simulink model "untitled_restored_from_autosave"  (R2025b)
settings: Solver=VariableStepAuto  StartTime=0.0  StopTime=40  RelTol=1e-3
values from neighbouring files (symbols this model uses):
  accel_bias = [0.05; 0.05; 0.05]    [init_sim_6dof.m]
  alt_bias = [0; 0; 15]    [init_sim_6dof.m]
  Cd_0 = [0.4, 0.42, 0.65, 0.55, 0.45, 0.35, 0.30, 0.28]    [init_sim_6dof.m]
  Cma = [-25, -28, -35,  -40,  -35,  -30,  -25,  -20 ]    [init_sim_6dof.m]
  Cme = -15    [init_sim_6dof.m]
  Cna = [15,  16,   18,   20,   18,   15,   12,   10  ]    [init_sim_6dof.m]
  Cne = -15    [init_sim_6dof.m]
  Empuje_Max = 16000    [init_sim_6dof.m]
  gyro_bias = [0.01; 0.01; 0.01]    [init_sim_6dof.m]
  L_ref = diametro    (= 0.127)    [init_sim_6dof.m]
  lat_0 = 40.4168    [init_sim_6dof.m]
  lon_0 = -3.7038    [init_sim_6dof.m]
  Mach_vec = [0.0, 0.8, 1.0, 1.2, 1.5, 2.0, 3.0, 4.0]    [init_sim_6dof.m]
  masa_ini = 85.0    (= 85)    [init_sim_6dof.m]
  N_pn = 4.0    (= 4)    [init_sim_6dof.m]
  pitch_0 = 0    [init_sim_6dof.m]
  pos_0_ned = [0; 0; -alt_0]    [init_sim_6dof.m]
  pos_target_0 = [10000; 0; -5000]    [init_sim_6dof.m]
  quat_0 = angle2quat(yaw_0, pitch_0, roll_0, 'ZYX')'    [init_sim_6dof.m]
  roll_0 = 0    [init_sim_6dof.m]
  S_ref = pi*(diametro/2)^2    (= 0.0126676869774)    [init_sim_6dof.m]
  t_burn = 5.0    (= 5)    [init_sim_6dof.m]
  Ts = 0.005    [init_sim_6dof.m]
  Ts_gnss = 0.1    [init_sim_6dof.m]
  vel_target_0 = [-250; 0; 0]    [init_sim_6dof.m]
  yaw_0 = 0    [init_sim_6dof.m]
undefined symbols (not defined in the file or in its folder): Accel_Body, magnitude, Omega_Body, Pos_NED
libraries: simulink x5, slpidlib x2, aerolibasang x2, aerolibanim x1, aerolibatmos2 x1
settings Model: Creator=Pc  LastModifiedBy=Pc

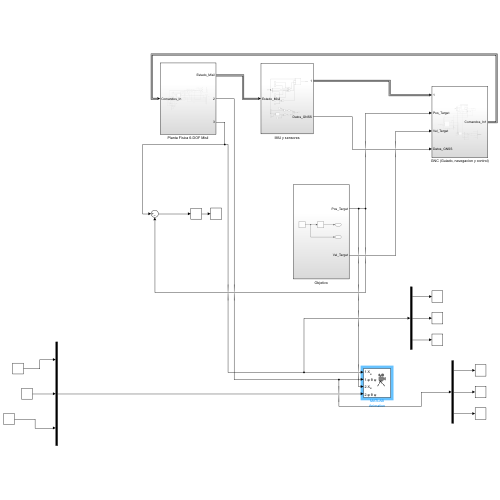
[thumbnail: Simulink's stored preview of the top-level diagram]
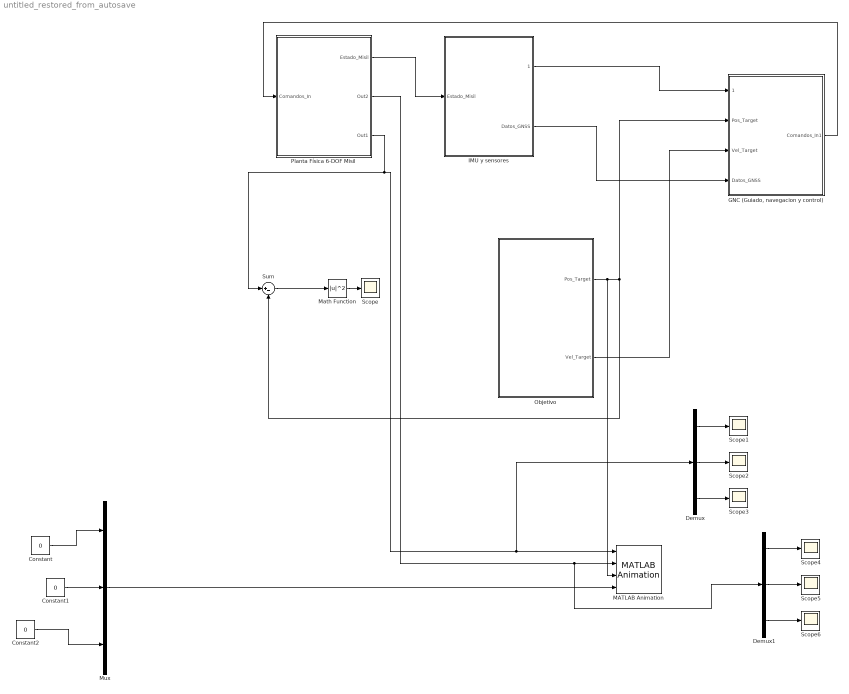
== system untitled_restored_from_autosave ==
  Constant : Constant  Value=0
  Constant1 : Constant  Value=0
  Constant2 : Constant  Value=0
  Demux : Demux  Outputs=3
  Demux1 : Demux  Outputs=3
  "GNC (Guiado, navegacion y control)" : Subsystem
  IMU y sensores : Subsystem
  MATLAB Animation : aerolibanim/MATLAB Animation  Tag=Matlab Animation 6 DOF  Vehicles=2  Geometries={'testrocket.ac', 'pa24-250_orange.ac'}  BoundingBoxCoordinates=[-50,50,-50,50,-50,50]  CameraOffset=[-150,-50,0]  CameraViewAngle=50  SampleTime=0.05  FigurePosition=[-248,-120,605,515]
  Math Function : Math  Operator=magnitude^2
  Mux : Mux  Inputs=3
  Objetivo : Subsystem
  Planta Física 6-DOF Misil : Subsystem
  Scope{,1..6} (7 alike) : Scope
      Scope settings: ActiveDisplayYMinimum=-2.9498159445716068E+7  ActiveDisplayYMaximum=4.0106517826440394E+7
      Scope1 settings: ActiveDisplayYMinimum=-21.388722849455736  ActiveDisplayYMaximum=29.150281058057079  DataLoggingVariableName=ScopeData2
      Scope2 settings: DataLoggingVariableName=ScopeData3
      Scope3 settings: ActiveDisplayYMinimum=-15.325503543946462  ActiveDisplayYMaximum=15.701060775623862  DataLoggingVariableName=ScopeData4
      Scope4 settings: ActiveDisplayYMinimum=-2.4693491349201278  ActiveDisplayYMaximum=1.7034269315097514  DataLoggingVariableName=ScopeData5
      Scope5 settings: ActiveDisplayYMinimum=-1.9297866797423937  ActiveDisplayYMaximum=2.0089780542618731  DataLoggingVariableName=ScopeData6
      Scope6 settings: ActiveDisplayYMinimum=-1  ActiveDisplayYMaximum=1  DataLoggingVariableName=ScopeData7
  Sum : Sum  Inputs=|+-
  wires:
  Planta Física 6-DOF Misil/1(Estado_Misil) -> IMU y sensores/1(Estado_Misil)
  IMU y sensores/1(1) -> "GNC (Guiado, navegacion y control)"/1(1)
  Objetivo/1(Pos_Target) -> MATLAB Animation/3, Sum/2, "GNC (Guiado, navegacion y control)"/2(Pos_Target)
  Objetivo/2(Vel_Target) -> "GNC (Guiado, navegacion y control)"/3(Vel_Target)
  "GNC (Guiado, navegacion y control)"/1(Comandos_In1) -> Planta Física 6-DOF Misil/1(Comandos_In)
  Sum/1 -> Math Function/1
  Math Function/1 -> Scope/1
  IMU y sensores/2(Datos_GNSS) -> "GNC (Guiado, navegacion y control)"/4(Datos_GNSS)
  Planta Física 6-DOF Misil/2(Out2) -> Demux1/1, MATLAB Animation/2
  Constant2/1 -> Mux/3
  Constant1/1 -> Mux/2
  Constant/1 -> Mux/1
  Mux/1 -> MATLAB Animation/4
  Planta Física 6-DOF Misil/3(Out1) -> Sum/1, Demux/1, MATLAB Animation/1
  Demux1/3 -> Scope6/1
  Demux1/2 -> Scope5/1
  Demux1/1 -> Scope4/1
  Demux/3 -> Scope3/1
  Demux/2 -> Scope2/1
  Demux/1 -> Scope1/1

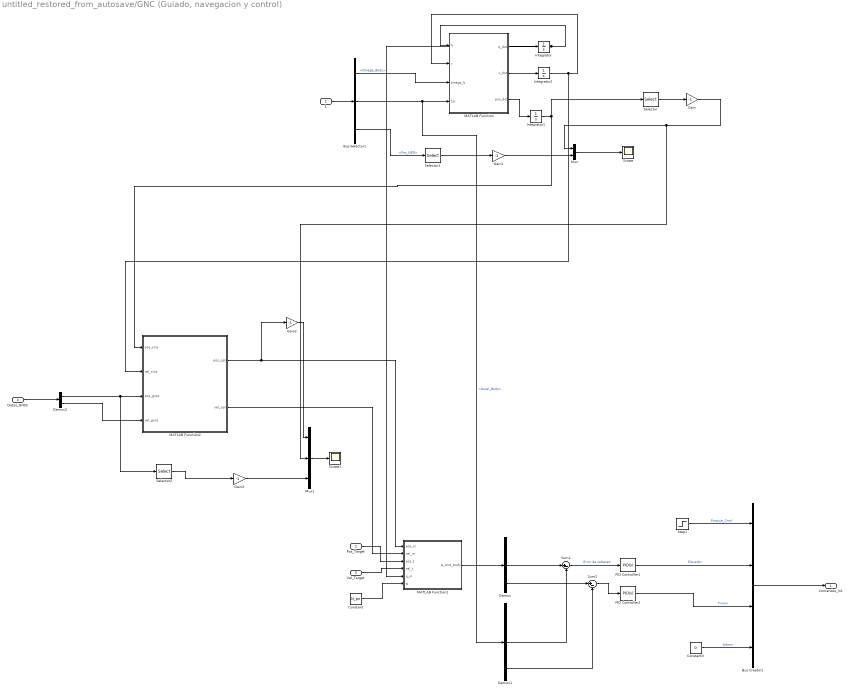
== system untitled_restored_from_autosave/GNC (Guiado, navegacion y control) ==
  1 : Inport  OutDataTypeStr=Bus: Bus_Estado
  Pos_Target : Inport  Port=2
  Vel_Target : Inport  Port=3
  Datos_GNSS : Inport  Port=4
  Bus Creator1 : BusCreator  Inputs=4  OutDataTypeStr=Bus: Bus_Comandos
  Bus Selector1 : BusSelector  OutputSignals=Omega_Body,Accel_Body,Pos_NED
  Constant : Constant  Value=N_pn
  Constant3 : Constant  Value=0
  Demux : Demux  Outputs=3
  Demux1 : Demux  Outputs=3
  Demux2 : Demux  Outputs=2
  Gain{,1..3} (4 alike) : Gain  Gain=-1
  Integrator : Integrator  InitialCondition=quat_0
  Integrator1 : Integrator  InitialCondition=pos_0_ned
  Integrator2 : Integrator  InitialCondition=[250; 0; 0]
  MATLAB Function : MATLAB Function  TreatAsAtomicUnit=on
  MATLAB Function1 : MATLAB Function  TreatAsAtomicUnit=on
  MATLAB Function2 : MATLAB Function  TreatAsAtomicUnit=on
  Mux : Mux  Inputs=2
  Mux1 : Mux  Inputs=3
  PID Controller1 : slpidlib/PID Controller  Controller=PID  Form=Parallel  TimeDomain=Continuous-time  UseExternalTs=off  SampleTime=-1  IntegratorMethod=Forward Euler  FilterMethod=Forward Euler  ControllerParametersSource=internal  P=0.05  I=0.01  UseKiTs=off  D=0  UseExternalDerivativeSource=off  N=100  UseFilter=on  TunerSelectOption=Transfer Function Based (PID Tuner App)  InitialConditionSource=internal  InitialConditionForIntegrator=0  InitialConditionForFilter=0  DifferentiatorICPrevScaledInput=0  ExternalReset=none  TrackingMode=off  Kt=1  LimitOutput=on  SatLimitsSource=internal  UpperSaturationLimit=0.5  LowerSaturationLimit=-0.5  LinearizeAsGain=on  AntiWindupMode=none  Kb=1  LimitIntegrator=off  UpperIntegratorSaturationLimit=inf  LowerIntegratorSaturationLimit=-inf  POutMin=[]  POutMax=[]  IOutMin=[]  IOutMax=[]  DOutMin=[]  DOutMax=[]  NOutMin=[]  NOutMax=[]  SumOutMin=[]  SumOutMax=[]  SaturationOutMin=[]  SaturationOutMax=[]  PParamMin=[]  PParamMax=[]  IParamMin=[]  IParamMax=[]  DParamMin=[]  DParamMax=[]  NParamMin=[]  NParamMax=[]  KbParamMin=[]  KbParamMax=[]  KtParamMin=[]  KtParamMax=[]  KbOutMin=[]  KbOutMax=[]  KtOutMin=[]  KtOutMax=[]  IntegratorOutMin=[]  IntegratorOutMax=[]  FilterOutMin=[]  FilterOutMax=[]  SumI1OutMin=[]  SumI1OutMax=[]  SumI2OutMin=[]  SumI2OutMax=[]  SumI3OutMin=[]  SumI3OutMax=[]  SumI4OutMin=[]  SumI4OutMax=[]  SumDOutMin=[]  SumDOutMax=[]  DifferentiatorOutMin=[]  DifferentiatorOutMax=[]  FilterDiffOutCoefMin=[]  FilterDiffOutCoefMax=[]  ReciprocalOutMin=[]  ReciprocalOutMax=[]  SumDenOutMin=[]  SumDenOutMax=[]  SumNumOutMin=[]  SumNumOutMax=[]  DivideOutMin=[]  DivideOutMax=[]  UdiffTsProdOutMin=[]  UdiffTsProdOutMax=[]  NTsProdOutMin=[]  NTsProdOutMax=[]  UintegralTsProdOutMin=[]  UintegralTsProdOutMax=[]  UngainTsProdOutMin=[]  UngainTsProdOutMax=[]  ClampingZeroOutDataTypeStr=Inherit: Inherit via back propagation  ClampingZeroOutMin=[]  ClampingZeroOutMax=[]  FilterDenConstantOutDataTypeStr=Inherit: Inherit via back propagation  FilterDenConstantOutMin=[]  FilterDenConstantOutMax=[]  PCopyOutDataTypeStr=Inherit: Inherit via back propagation  PCopyOutMin=[]  PCopyOutMax=[]  NCopyOutDataTypeStr=Inherit: Inherit via back propagation  NCopyOutMin=[]  NCopyOutMax=[]  IntegratorContinuousStateAttributes=''  IntegratorStateMustResolveToSignalObject=off  IntegratorRTWStateStorageClass=Auto  FilterContinuousStateAttributes=''  FilterStateMustResolveToSignalObject=off  FilterRTWStateStorageClass=Auto  ParallelPVariant=InternalParameters  IdealPVariant=Disabled  IVariant=InternalParameters  DVariant=InternalParameters  IntegratorVariant=Continuous  SatVariant=Enabled  AWVariant=Passthrough  PCopyVariant=Disabled  TRVariant=Disabled  FdbkBlocksVariant=Forward  IdealPFdbkVariant=Disabled  SatFdbkVariant=Disabled  DerivativeFilterVariant=ContFilter  NVariant=InternalParameters  NCopyVariant=Disabled  FilterICVariant=InternalICsFilter  IntegratorICVariant=InternalICs  ExternalResetVariant=Disabled  TRSumVariant=Passthrough  SumFdbkVariant=Disabled  SumVariant=Sum_PID  TsampFilterVariant=InternalTs  TsampNgainVariant=Passthrough  TsampIntegralVariant=Disabled_SignalSpec  ExternalSaturationOutDataTypeStr=Inherit: Same as second input  DerivativeSourceVariant=ErrorSignal  PreIntVariant=InternalPreInt
  PID Controller2 : slpidlib/PID Controller  Controller=PID  Form=Parallel  TimeDomain=Continuous-time  UseExternalTs=off  SampleTime=-1  IntegratorMethod=Forward Euler  FilterMethod=Forward Euler  ControllerParametersSource=internal  P=0.05  I=0.01  UseKiTs=off  D=0  UseExternalDerivativeSource=off  N=100  UseFilter=on  TunerSelectOption=Transfer Function Based (PID Tuner App)  InitialConditionSource=internal  InitialConditionForIntegrator=0  InitialConditionForFilter=0  DifferentiatorICPrevScaledInput=0  ExternalReset=none  TrackingMode=off  Kt=1  LimitOutput=on  SatLimitsSource=internal  UpperSaturationLimit=0.5  LowerSaturationLimit=-0.5  LinearizeAsGain=on  AntiWindupMode=none  Kb=1  LimitIntegrator=off  UpperIntegratorSaturationLimit=inf  LowerIntegratorSaturationLimit=-inf  POutMin=[]  POutMax=[]  IOutMin=[]  IOutMax=[]  DOutMin=[]  DOutMax=[]  NOutMin=[]  NOutMax=[]  SumOutMin=[]  SumOutMax=[]  SaturationOutMin=[]  SaturationOutMax=[]  PParamMin=[]  PParamMax=[]  IParamMin=[]  IParamMax=[]  DParamMin=[]  DParamMax=[]  NParamMin=[]  NParamMax=[]  KbParamMin=[]  KbParamMax=[]  KtParamMin=[]  KtParamMax=[]  KbOutMin=[]  KbOutMax=[]  KtOutMin=[]  KtOutMax=[]  IntegratorOutMin=[]  IntegratorOutMax=[]  FilterOutMin=[]  FilterOutMax=[]  SumI1OutMin=[]  SumI1OutMax=[]  SumI2OutMin=[]  SumI2OutMax=[]  SumI3OutMin=[]  SumI3OutMax=[]  SumI4OutMin=[]  SumI4OutMax=[]  SumDOutMin=[]  SumDOutMax=[]  DifferentiatorOutMin=[]  DifferentiatorOutMax=[]  FilterDiffOutCoefMin=[]  FilterDiffOutCoefMax=[]  ReciprocalOutMin=[]  ReciprocalOutMax=[]  SumDenOutMin=[]  SumDenOutMax=[]  SumNumOutMin=[]  SumNumOutMax=[]  DivideOutMin=[]  DivideOutMax=[]  UdiffTsProdOutMin=[]  UdiffTsProdOutMax=[]  NTsProdOutMin=[]  NTsProdOutMax=[]  UintegralTsProdOutMin=[]  UintegralTsProdOutMax=[]  UngainTsProdOutMin=[]  UngainTsProdOutMax=[]  ClampingZeroOutDataTypeStr=Inherit: Inherit via back propagation  ClampingZeroOutMin=[]  ClampingZeroOutMax=[]  FilterDenConstantOutDataTypeStr=Inherit: Inherit via back propagation  FilterDenConstantOutMin=[]  FilterDenConstantOutMax=[]  PCopyOutDataTypeStr=Inherit: Inherit via back propagation  PCopyOutMin=[]  PCopyOutMax=[]  NCopyOutDataTypeStr=Inherit: Inherit via back propagation  NCopyOutMin=[]  NCopyOutMax=[]  IntegratorContinuousStateAttributes=''  IntegratorStateMustResolveToSignalObject=off  IntegratorRTWStateStorageClass=Auto  FilterContinuousStateAttributes=''  FilterStateMustResolveToSignalObject=off  FilterRTWStateStorageClass=Auto  ParallelPVariant=InternalParameters  IdealPVariant=Disabled  IVariant=InternalParameters  DVariant=InternalParameters  IntegratorVariant=Continuous  SatVariant=Enabled  AWVariant=Passthrough  PCopyVariant=Disabled  TRVariant=Disabled  FdbkBlocksVariant=Forward  IdealPFdbkVariant=Disabled  SatFdbkVariant=Disabled  DerivativeFilterVariant=ContFilter  NVariant=InternalParameters  NCopyVariant=Disabled  FilterICVariant=InternalICsFilter  IntegratorICVariant=InternalICs  ExternalResetVariant=Disabled  TRSumVariant=Passthrough  SumFdbkVariant=Disabled  SumVariant=Sum_PID  TsampFilterVariant=InternalTs  TsampNgainVariant=Passthrough  TsampIntegralVariant=Disabled_SignalSpec  ExternalSaturationOutDataTypeStr=Inherit: Same as second input  DerivativeSourceVariant=ErrorSignal  PreIntVariant=InternalPreInt
  Scope : Scope
      settings: ActiveDisplayYMinimum=-3409.6489857780471  ActiveDisplayYMaximum=9919.0359935642336
  Scope1 : Scope
      settings: ActiveDisplayYMinimum=-14494.057795394729  ActiveDisplayYMaximum=13064.034716970949
  Selector : Selector  InputPortWidth=3  IndexOptions=Index vector (dialog)  Indices=3  OutputSizes=1
  Selector1 : Selector  InputPortWidth=3  IndexOptions=Index vector (dialog)  Indices=3  OutputSizes=1
  Selector2 : Selector  InputPortWidth=3  IndexOptions=Index vector (dialog)  Indices=3  OutputSizes=1
  Step1 : Step  Time=t_burn  Before=Empuje_Max  After=0  SampleTime=0
  Sum1 : Sum  Inputs=|+-
  Sum2 : Sum  Inputs=|+-
  Comandos_In1 : Outport
  wires:
  Selector/1 -> Gain/1
  Gain/1 -> Mux1/2, Mux/1
  1/1 -> Bus Selector1/1
  MATLAB Function/1(q_dot) -> Integrator/1
  MATLAB Function/2(v_dot) -> Integrator2/1
  MATLAB Function/3(pos_dot) -> Integrator1/1
  Integrator/1 -> MATLAB Function/1(q), MATLAB Function1/5(q_m)
  Integrator2/1 -> MATLAB Function2/2(vel_sins), MATLAB Function/2(v)
  Bus Selector1/1 -> MATLAB Function/3(omega_b)  "<Omega_Body>"
  Bus Selector1/2 -> Demux1/1, MATLAB Function/4(f_b)  "<Accel_Body>"
  Integrator1/1 -> Selector/1, MATLAB Function2/1(pos_sins)
  Gain1/1 -> Mux/2
  Selector1/1 -> Gain1/1
  Bus Selector1/3 -> Selector1/1  "<Pos_NED>"
  Mux/1 -> Scope/1
  Pos_Target/1 -> MATLAB Function1/3(pos_t)
  Vel_Target/1 -> MATLAB Function1/4(vel_t)
  Constant/1 -> MATLAB Function1/6(N)
  MATLAB Function1/1(A_cmd_body) -> Demux/1
  Demux/2 -> Sum1/1
  Demux1/2 -> Sum1/2
  Sum1/1 -> PID Controller1/1  "Error de cabeceo"
  PID Controller1/1 -> Bus Creator1/2  "Elevador"
  Demux/3 -> Sum2/1
  Demux1/3 -> Sum2/2
  Sum2/1 -> PID Controller2/1
  PID Controller2/1 -> Bus Creator1/3  "Timon"
  Step1/1 -> Bus Creator1/1  "Empuje_Cmd"
  Constant3/1 -> Bus Creator1/4  "Aleron"
  Bus Creator1/1 -> Comandos_In1/1
  Datos_GNSS/1 -> Demux2/1
  Demux2/1 -> Selector2/1, MATLAB Function2/3(pos_gnss)
  Demux2/2 -> MATLAB Function2/4(vel_gnss)
  MATLAB Function2/1(pos_opt) -> Gain2/1, MATLAB Function1/1(pos_m)
  MATLAB Function2/2(vel_opt) -> MATLAB Function1/2(vel_m)
  Gain2/1 -> Mux1/1
  Mux1/1 -> Scope1/1
  Selector2/1 -> Gain3/1
  Gain3/1 -> Mux1/3

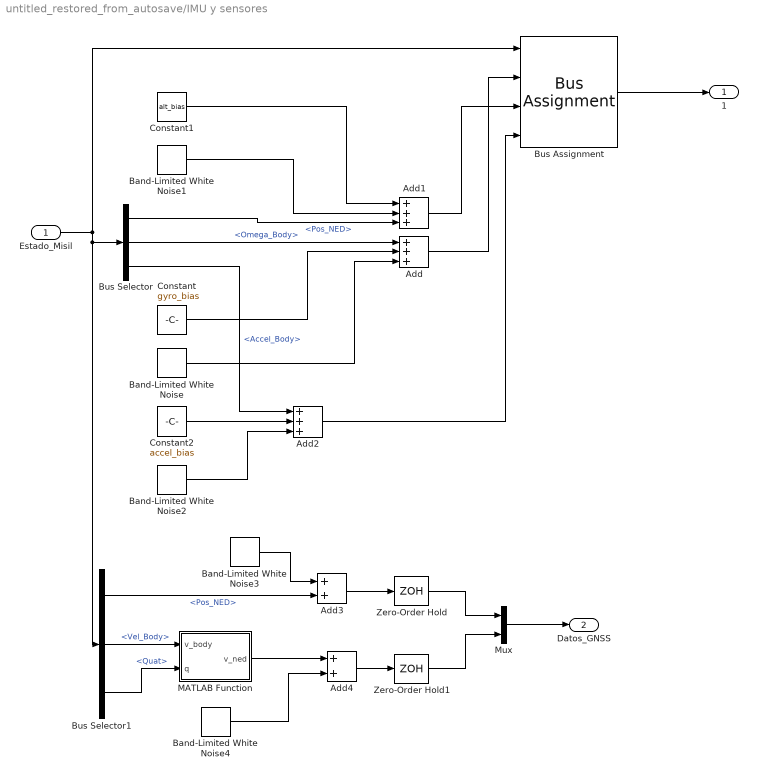
== system untitled_restored_from_autosave/IMU y sensores ==
  Estado_Misil : Inport  OutDataTypeStr=Bus: Bus_Estado
  Add : Sum  Inputs=+++
  Add1 : Sum  Inputs=+++
  Add2 : Sum  Inputs=+++
  Add3 : Sum
  Add4 : Sum
  Band-Limited White Noise : simulink/Sources/Band-Limited White Noise  Cov=gyro_noise_power  Ts=Ts  seed=[23341]
  Band-Limited White Noise1 : simulink/Sources/Band-Limited White Noise  Cov=alt_noise_power  Ts=Ts  seed=[23341]
  Band-Limited White Noise2 : simulink/Sources/Band-Limited White Noise  Cov=accel_noise_power  Ts=Ts  seed=[23341]
  Band-Limited White Noise3 : simulink/Sources/Band-Limited White Noise  Cov=gnss_noise_pos  Ts=Ts_gnss  seed=[23341]
  Band-Limited White Noise4 : simulink/Sources/Band-Limited White Noise  Cov=gnss_noise_vel  Ts=Ts_gnss  seed=[23341]
  Bus Assignment : BusAssignment  AssignedSignals=Omega_Body,Pos_NED,Accel_Body
  Bus Selector : BusSelector  OutputSignals=Pos_NED,Omega_Body,Accel_Body
  Bus Selector1 : BusSelector  OutputSignals=Pos_NED,Vel_Body,Quat
  Constant : Constant  Value=gyro_bias
  Constant1 : Constant  Value=alt_bias
  Constant2 : Constant  Value=accel_bias
  MATLAB Function : MATLAB Function  TreatAsAtomicUnit=on
  Mux : Mux  Inputs=2
  Zero-Order Hold : ZeroOrderHold  SampleTime=Ts_gnss
  Zero-Order Hold1 : ZeroOrderHold  SampleTime=Ts_gnss
  1 : Outport  OutDataTypeStr=Bus: Bus_Estado
  Datos_GNSS : Outport  Port=2
  wires:
  Bus Selector/2 -> Add/1  "<Omega_Body>"
  Constant/1 -> Add/2
  Band-Limited White Noise/1 -> Add/3
  Bus Selector/1 -> Add1/3  "<Pos_NED>"
  Band-Limited White Noise1/1 -> Add1/2
  Constant1/1 -> Add1/1
  Add/1 -> Bus Assignment/2
  Add1/1 -> Bus Assignment/3
  Bus Assignment/1 -> 1/1
  Bus Selector/3 -> Add2/1  "<Accel_Body>"
  Constant2/1 -> Add2/2
  Band-Limited White Noise2/1 -> Add2/3
  Add2/1 -> Bus Assignment/4
  Estado_Misil/1 -> Bus Selector1/1, Bus Selector/1, Bus Assignment/1
  Bus Selector1/2 -> MATLAB Function/1(v_body)  "<Vel_Body>"
  Bus Selector1/3 -> MATLAB Function/2(q)  "<Quat>"
  Bus Selector1/1 -> Add3/2  "<Pos_NED>"
  Band-Limited White Noise3/1 -> Add3/1
  Add3/1 -> Zero-Order Hold/1
  Add4/1 -> Zero-Order Hold1/1
  MATLAB Function/1(v_ned) -> Add4/1
  Band-Limited White Noise4/1 -> Add4/2
  Zero-Order Hold/1 -> Mux/1
  Zero-Order Hold1/1 -> Mux/2
  Mux/1 -> Datos_GNSS/1

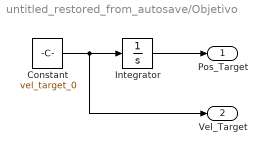
== system untitled_restored_from_autosave/Objetivo ==
  Constant : Constant  Value=vel_target_0
  Integrator : Integrator  InitialCondition=pos_target_0
  Pos_Target : Outport
  Vel_Target : Outport  Port=2
  wires:
  Constant/1 -> Vel_Target/1, Integrator/1
  Integrator/1 -> Pos_Target/1

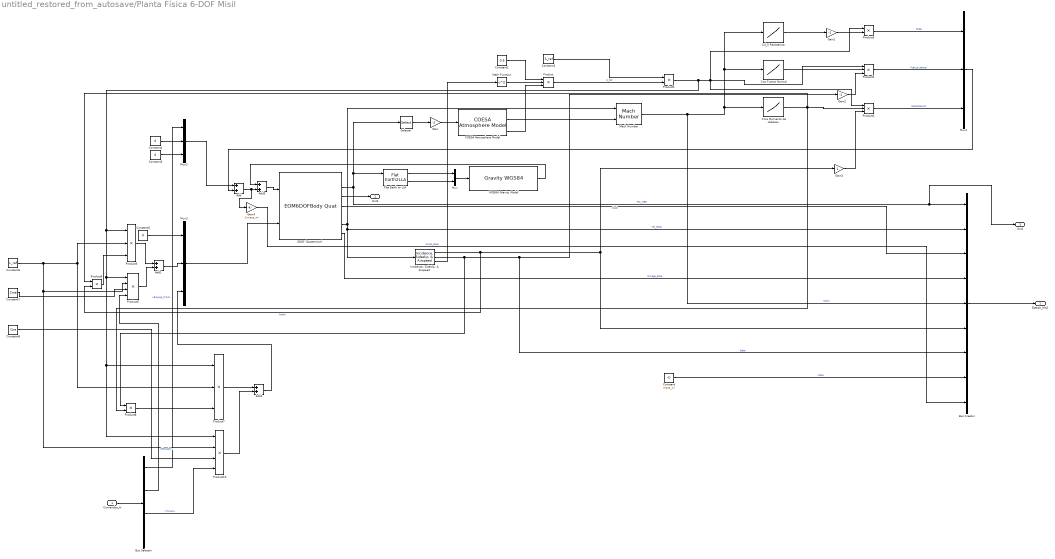
== system untitled_restored_from_autosave/Planta Física 6-DOF Misil ==
  Comandos_In : Inport  OutDataTypeStr=Bus: Bus_Comandos
  6DOF (Quaternion) : EOM6DOFBodyQuat  xme_0=pos_0_ned  Vm_0=vel_0_body  eul_0=[roll_0, pitch_0, yaw_0]  pm_0=omega_0_body  mass_0=masa_ini  inertia=I_tensor
  Add{,1..3} (4 alike) : Sum
  Bus Creator : BusCreator  Inputs=9  OutDataTypeStr=Bus: Bus_Estado
  Bus Selector : BusSelector  OutputSignals=Empuje_Cmd,Elevador,Timon,Aleron
  COESA Atmosphere Model : aerolibatmos2/COESA Atmosphere Model  units=Metric (MKS)  spec=1976 COESA-extended U.S. Standard Atmosphere  model=Profile  profile_var=High temperature  profile_percent=1%  profile_alt=5 km (16404 ft)  envelope_var=High temperature  envelope_percent=1%  action=Warning
  Cd_0 Resistencia : Lookup_n-D  NumberOfTableDimensions=1  BreakpointsForDimension1=Mach_vec  Table=Cd_0  InternalRulePriority=Speed  RndMeth=Simplest
  Cma Momento de cabeceo : Lookup_n-D  NumberOfTableDimensions=1  BreakpointsForDimension1=Mach_vec  Table=Cma  InternalRulePriority=Speed  RndMeth=Simplest
  Cna Fuerza Normal : Lookup_n-D  NumberOfTableDimensions=1  BreakpointsForDimension1=Mach_vec  Table=Cna  InternalRulePriority=Speed  RndMeth=Simplest
  Constant : Constant  Value=masa_ini
  Constant1 : Constant  Value=0.5
  Constant2 : Constant  Value=S_ref
  Constant3 : Constant  Value=0
  Constant4 : Constant  Value=0
  Constant5 : Constant  Value=0
  Constant6 : Constant  Value=L_ref
  Constant7 : Constant  Value=Cme
  Constant8 : Constant  Value=Cne
  Flat Earth to LLA : FlatEarth2LLA  LL0=[lat_0 lon_0]
  Gain : Gain  Gain=-1
  Gain1 : Gain  Gain=-1
  Gain2 : Gain  Gain=-1
  Gain3 : Gain
  Gain4 : Gain  Gain=1/masa_ini
  "Incidence, Sideslip, & Airspeed" : aerolibasang/Incidence, Sideslip, & Airspeed
  Mach Number : aerolibasang/Mach Number
  Math Function : Math  Operator=square
  Mux : Mux  Inputs=2
  Mux1 : Mux  Inputs=3
  Mux2 : Mux  Inputs=3
  Mux3 : Mux  Inputs=3
  Product{,2,4..5,7} (5 alike) : Product  Inputs=3
  Product{1,3,6,8} (4 alike) : Product
  Product10 : Product  Inputs=4
  Product9 : Product  Inputs=4
  Selector : Selector  InputPortWidth=3  IndexOptions=Index vector (dialog)  Indices=3  OutputSizes=1
  "WGS84 Gravity Model  " : GravityWGS84
  Estado_Misil : Outport  OutDataTypeStr=Bus: Bus_Estado
  Out2 : Outport  Port=2
  Out1 : Outport  Port=3
  wires:
  6DOF (Quaternion)/2 -> Out1/1, Bus Creator/1, Selector/1, Flat Earth to LLA/1  "Pos_NED"
  Selector/1 -> Gain/1
  Gain/1 -> COESA Atmosphere Model/1
  Flat Earth to LLA/1 -> Mux/1
  Flat Earth to LLA/2 -> Mux/2
  Mux/1 -> "WGS84 Gravity Model  "/1
  6DOF (Quaternion)/6 -> "Incidence, Sideslip, & Airspeed"/1, Bus Creator/2, Mach Number/1  "Vel_Body"
  COESA Atmosphere Model/2 -> Mach Number/2
  6DOF (Quaternion)/4 -> Bus Creator/3  "Quat"
  6DOF (Quaternion)/7 -> Bus Creator/4  "Omega_Body"
  Mach Number/1 -> Cma Momento de cabeceo/1, Cd_0 Resistencia/1, Cna Fuerza Normal/1, Bus Creator/5  "Mach"
  "Incidence, Sideslip, & Airspeed"/1 -> Product6/2, Gain3/1, Bus Creator/6  "Alpha"
  "Incidence, Sideslip, & Airspeed"/2 -> Product8/1, Gain2/1, Bus Creator/7  "Beta"
  Constant/1 -> Bus Creator/8  "Masa"
  "Incidence, Sideslip, & Airspeed"/3 -> Math Function/1
  Constant1/1 -> Product/1
  Math Function/1 -> Product/2
  COESA Atmosphere Model/4 -> Product/3
  Constant2/1 -> Product1/1
  Product/1 -> Product1/2  "q_bar"
  Cd_0 Resistencia/1 -> Gain1/1
  Product1/1 -> Product10/1, Product7/1, Product9/1, Product5/1, Product4/1, Product3/1, Product2/1
  Cna Fuerza Normal/1 -> Product2/2
  Gain2/1 -> Product2/3
  Gain1/1 -> Product3/2
  Cma Momento de cabeceo/1 -> Product8/2, Product6/1, Product4/2
  Gain3/1 -> Product4/3
  Product2/1 -> Mux1/2  "Fuerza Lateral"
  Product3/1 -> Mux1/1  "Drag"
  Product4/1 -> Mux1/3  "Sustentación"
  Constant4/1 -> Mux2/2
  Constant3/1 -> Mux2/3
  Mux1/1 -> Add/2
  Constant5/1 -> Mux3/1
  Constant6/1 -> Product10/2, Product9/2, Product7/2, Product5/2
  Product6/1 -> Product5/3
  Product8/1 -> Product7/3
  Mux3/1 -> 6DOF (Quaternion)/2
  Comandos_In/1 -> Bus Selector/1
  Bus Selector/1 -> Mux2/1  "<Empuje_Cmd>"
  Product5/1 -> Add1/1
  Add1/1 -> Mux3/2
  Constant7/1 -> Product9/3
  Bus Selector/2 -> Product9/4  "<Elevador>"
  Product9/1 -> Add1/2
  Product7/1 -> Add2/1
  Add2/1 -> Mux3/3
  Constant8/1 -> Product10/3
  Bus Selector/3 -> Product10/4  "<Timon>"
  Product10/1 -> Add2/2
  Mux2/1 -> Add/1
  Add/1 -> Gain4/1, Add3/2
  Add3/1 -> 6DOF (Quaternion)/1
  "WGS84 Gravity Model  "/1 -> Add3/1
  Gain4/1 -> Bus Creator/9  "Accel_Body"
  Bus Creator/1 -> Estado_Misil/1
  6DOF (Quaternion)/3 -> Out2/1

== matlab function untitled_restored_from_autosave/GNC (Guiado, navegacion y control)/MATLAB Function1 ==
  data: pos_m input; A_cmd_body output; vel_m input; pos_t input; vel_t input; q_m input; N input
function A_cmd_body  = guiado_pn(pos_m, vel_m, pos_t, vel_t, q_m, N)
    % 1. Cinemática Relativa
    R_vec = pos_t - pos_m;            
    V_rel = vel_t - vel_m;            
    r = norm(R_vec);                  
    
    if r < 1
        A_cmd_body = [0; 0; 0];
        return;
    end
    
    % 2. Línea de Visión y Velocidad de Cierre
    lambda = R_vec / r;               
    Vc = -dot(R_vec, V_rel) / r; 
    Omega_LOS = cross(R_vec, V_rel) / (r^2);
    
    % 3. Ley PN en ejes NED
    A_cmd_ned = N * Vc * cross(Omega_LOS, lambda);
    
    % 4. TRADUCTOR: Rotación a Ejes Cuerpo (NED -> Body)
    q0 = q_m(1); q1 = q_m(2); q2 = q_m(3); q3 = q_m(4);
    C_n_b = [q0^2+q1^2-q2^2-q3^2,     2*(q1*q2+q0*q3),     2*(q1*q3-q0*q2);
             2*(q1*q2-q0*q3),         q0^2-q1^2+q2^2-q3^2, 2*(q2*q3+q0*q1);
             2*(q1*q3+q0*q2),         2*(q2*q3-q0*q1),     q0^2-q1^2-q2^2+q3^2];
             
    A_cmd_body = C_n_b * A_cmd_ned;
end

== matlab function untitled_restored_from_autosave/GNC (Guiado, navegacion y control)/MATLAB Function ==
  data: q input; q_dot output; v input; omega_b input; f_b input; v_dot output; pos_dot output
function [q_dot, v_dot, pos_dot] = mecanizacion_sins(q, v, omega_b, f_b)
    % 1. EXTRACCIÓN DE DATOS
    p = omega_b(1); q_gy = omega_b(2); r = omega_b(3); % Tasas de giro
    q0 = q(1); q1 = q(2); q2 = q(3); q3 = q(4);        % Cuaternión (Escalar primero)
    
    % 2. ECUACIÓN DE ACTITUD (Derivada del Cuaternión)
    % Matriz antisimétrica de velocidades angulares
    Omega = [ 0,  -p,  -q_gy, -r;
              p,   0,   r,  -q_gy;
              q_gy, -r,   0,   p;
              r,   q_gy, -p,   0 ];
    q_dot = 0.5 * Omega * q;
    
    % 3. MATRIZ DE COSENOS DIRECTORES (DCM: Body -> NED)
    % Transforma vectores del misil a los ejes de la Tierra
    C_b_n = [q0^2+q1^2-q2^2-q3^2, 2*(q1*q2-q0*q3),     2*(q1*q3+q0*q2);
             2*(q1*q2+q0*q3),     q0^2-q1^2+q2^2-q3^2, 2*(q2*q3-q0*q1);
             2*(q1*q3-q0*q2),     2*(q2*q3+q0*q1),     q0^2-q1^2-q2^2+q3^2];
         
    % 4. ECUACIÓN DE VELOCIDAD (Aceleración Cinemática)
    g = 9.80665; % Gravedad local [m/s^2]
    % La derivada de la velocidad es la fuerza específica rotada a NED + la Gravedad
    v_dot = C_b_n * f_b + [0; 0; g];
    
    % 5. ECUACIÓN DE POSICIÓN
    pos_dot = v;
end

== matlab function untitled_restored_from_autosave/GNC (Guiado, navegacion y control)/MATLAB Function2 ==
  settings: updateMethod=DISCRETE
  data: pos_sins input; pos_opt output; vel_sins input; pos_gnss input; vel_gnss input; vel_opt output
function [pos_opt, vel_opt] = eskf_fusion(pos_sins, vel_sins, pos_gnss, vel_gnss)
    % Filtro de Kalman de Estados de Error (ESKF)
    % Mantiene la memoria del filtro entre ejecuciones
    persistent P delta_x last_pos_gnss

    % Inicialización (Solo ocurre en el t=0)
    if isempty(P)
        P = eye(6) * 10;          % Incertidumbre inicial
        delta_x = zeros(6,1);     % Error estimado inicial (asumimos 0)
        last_pos_gnss = [0;0;0];
    end

    dt = 0.01; % Tiempo de muestreo del GNC (Cámbialo si tu paso de Simulink es otro)

    % ---------------------------------------------------------
    % 1. PREDICCIÓN (El error del SINS crece con el tiempo)
    % ---------------------------------------------------------
    F = [eye(3), eye(3)*dt;
         zeros(3), eye(3)];
    Q = diag([1e-4, 1e-4, 1e-4, 1e-3, 1e-3, 1e-3]); % Ruido de proceso (Deriva IMU)

    delta_x = F * delta_x;
    P = F * P * F' + Q;

    % ---------------------------------------------------------
    % 2. ACTUALIZACIÓN (Solo cuando el GPS manda un dato nuevo)
    % ---------------------------------------------------------
    % Comprobamos si el GNSS ha cambiado (se actualiza más lento)
    if norm(pos_gnss - last_pos_gnss) > 1e-5
        last_pos_gnss = pos_gnss;

        % La "Medida" (z) es la diferencia entre SINS y GNSS
        z = [pos_sins - pos_gnss;
             vel_sins - vel_gnss];

        H = eye(6); % Observamos el error directamente
        R = diag([2, 2, 3, 0.1, 0.1, 0.15].^2); % Varianza del ruido GPS (del script)

        % Ecuaciones mágicas de Kalman
        S = H * P * H' + R;
        K = P * H' / S; % Ganancia de Kalman

        % Corregimos nuestra estimación del error
        delta_x = delta_x + K * (z - H * delta_x);

        % Actualizamos la matriz de covarianza
        P = (eye(6) - K * H) * P;
    end

    % ---------------------------------------------------------
    % 3. CORRECCIÓN FINAL
    % ---------------------------------------------------------
    % A la posición rápida del SINS le restamos el error estimado por Kalman
    pos_opt = pos_sins - delta_x(1:3);
    vel_opt = vel_sins - delta_x(4:6);
end

== matlab function untitled_restored_from_autosave/IMU y sensores/MATLAB Function ==
  data: v_body input; v_ned output; q input
function v_ned = body2ned(v_body, q)
    % Extraemos los componentes del cuaternión
    q0 = q(1); q1 = q(2); q2 = q(3); q3 = q(4);
    
    % Matriz de rotación de Cuerpo a Tierra (C_b_n)
    C_b_n = [q0^2+q1^2-q2^2-q3^2,     2*(q1*q2-q0*q3),     2*(q1*q3+q0*q2);
             2*(q1*q2+q0*q3),         q0^2-q1^2+q2^2-q3^2, 2*(q2*q3-q0*q1);
             2*(q1*q3-q0*q2),         2*(q2*q3+q0*q1),     q0^2-q1^2-q2^2+q3^2];
             
    % Rotamos la velocidad
    v_ned = C_b_n * v_body;
end
